simulink model "control_unstable"  (R2023b)
settings: Solver=VariableStepAuto  StartTime=0.0  StopTime=100  RelTol=1e-3
undefined symbols (not defined in the file): DiscIntNeverNeededParam
libraries: simulink x1
settings Model: Creator=awcm9  LastModifiedBy=awcm9

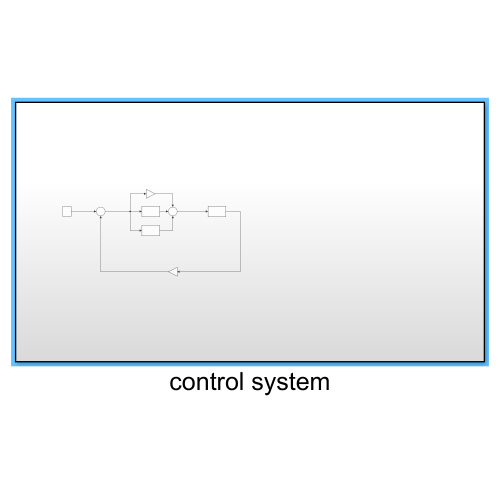
[thumbnail: Simulink's stored preview of the top-level diagram]
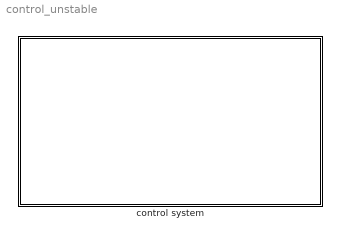
== system control_unstable ==
  control system : Subsystem

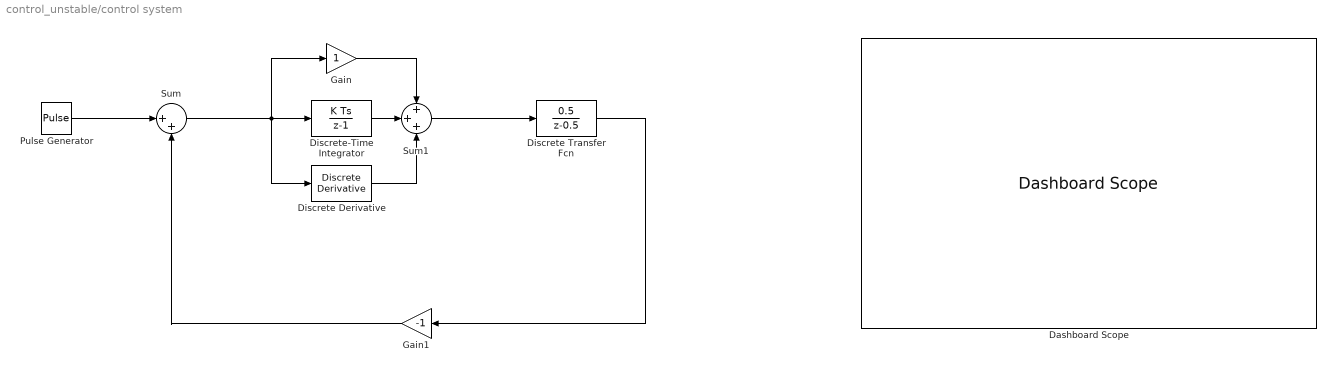
== system control_unstable/control system ==
  Dashboard Scope : DashboardScope  ShowInitialText=off  TimeSpan=20  Ymin=-1.0  Ymax=2.0  ScaleAtStop=off
  Discrete Transfer Fcn : DiscreteTransferFcn  Numerator=[0.5]  Denominator=[1 -0.5]
  Discrete Derivative : simulink/Discrete/Discrete Derivative  gainval=0.1  ICPrevScaledInput=0.0  OutMin=[]  OutMax=[]  OutDataType=fixdt(1, 16)  OutScaling=2^-10  DoSatur=off
  Discrete-Time Integrator : DiscreteIntegrator  gainval=1.5  SampleTime=-1  ICPrevOutput=DiscIntNeverNeededParam  ICPrevScaledInput=DiscIntNeverNeededParam
  Gain : Gain
  Gain1 : Gain  Gain=-1
  Pulse Generator : DiscretePulseGenerator  Period=20  PulseWidth=10
  Sum : Sum  Inputs=|++
  Sum1 : Sum  Inputs=+++
  wires:
  Gain1/1 -> Sum/2
  Discrete Derivative/1 -> Sum1/3
  Discrete-Time Integrator/1 -> Sum1/2
  Sum1/1 -> Discrete Transfer Fcn/1
  Gain/1 -> Sum1/1
  Discrete Transfer Fcn/1 -> Gain1/1
  Sum/1 -> Discrete-Time Integrator/1, Discrete Derivative/1, Gain/1
  Pulse Generator/1 -> Sum/1
